simulink model "SimulacaoEspacoEstadosExemplo"  (R2023a)
settings: Solver=VariableStepAuto  StartTime=0.0  StopTime=3  RelTol=1e-3
values from neighbouring files (symbols this model uses):
  A = [0 1; -K/M -b/M]    [ProjetoEspacoEstadosExemplo.m]    (also in ProjetoStateSpace.m = [-1 3; -2 -3])
  B = [0; 1/M]    [ProjetoEspacoEstadosExemplo.m]    (also in ProjetoStateSpace.m = [0; 5])
  h = double(Kras.H(1))    [ProjetoEspacoEstadosExemplo.m]
  k1 = double(Kras.K1(1))    [ProjetoEspacoEstadosExemplo.m]    (also in ProjetoStateSpace.m = sym('k1'))
  k2 = double(Kras.K2(1))    [ProjetoEspacoEstadosExemplo.m]    (also in ProjetoStateSpace.m = sym('k2'))
  Kreg = place(A,B,polosreg)    [ProjetoEspacoEstadosExemplo.m]
settings Model: Creator=a2270340  LastModifiedBy=a2270340

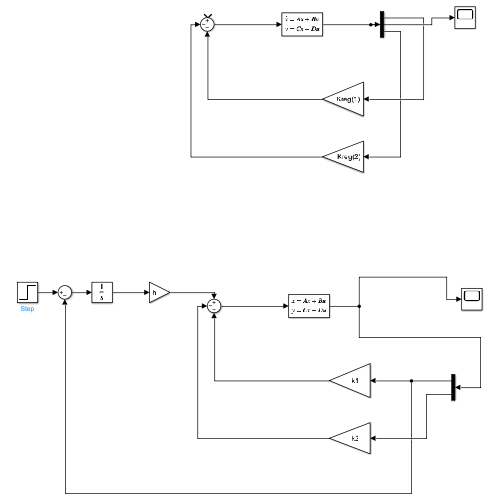
[thumbnail: Simulink's stored preview of the top-level diagram]
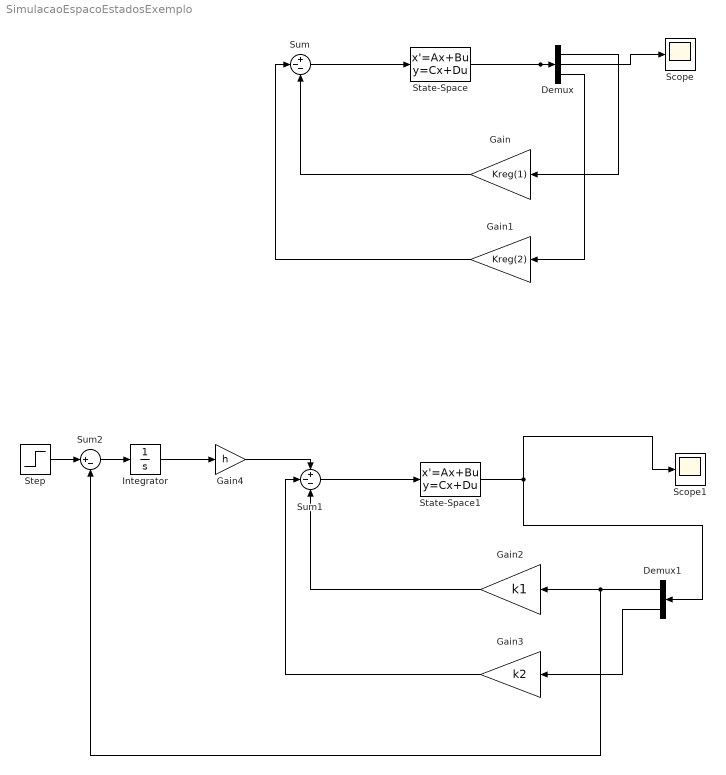
== system SimulacaoEspacoEstadosExemplo ==
  Demux : Demux  Outputs=2
  Demux1 : Demux  Outputs=2
  Gain : Gain  Gain=Kreg(1)
  Gain1 : Gain  Gain=Kreg(2)
  Gain2 : Gain  Gain=k1
  Gain3 : Gain  Gain=k2
  Gain4 : Gain  Gain=h
  Integrator : Integrator
  Scope : Scope
  Scope1 : Scope
  State-Space : StateSpace  A=A  B=B  C=[1 0; 0 1]  D=[0;0]  InitialCondition=[25;10]
  State-Space1 : StateSpace  A=A  B=B  C=[1 0; 0 1]  D=[0;0]  InitialCondition=0
  Step : Step  SampleTime=0
  Sum : Sum  Inputs=+--
  Sum1 : Sum  Inputs=+--
  Sum2 : Sum  Inputs=|+-
  wires:
  Sum/1 -> State-Space/1
  State-Space/1 -> Scope/1, Demux/1
  Demux/1 -> Gain/1
  Demux/2 -> Gain1/1
  Gain/1 -> Sum/3
  Gain1/1 -> Sum/2
  Gain2/1 -> Sum1/3
  State-Space1/1 -> Scope1/1, Demux1/1
  Gain3/1 -> Sum1/2
  Demux1/1 -> Sum2/2, Gain2/1
  Sum1/1 -> State-Space1/1
  Demux1/2 -> Gain3/1
  Sum2/1 -> Integrator/1
  Step/1 -> Sum2/1
  Integrator/1 -> Gain4/1
  Gain4/1 -> Sum1/1
